simulink model "chloro_m"  (Simulink 7.9)
settings: Solver=ode45  SolverMode=SingleTasking  StartTime=0.0  StopTime=999999  MaxStep=10  RelTol=1e-3  AbsTol=1e-3
values from neighbouring files (symbols this model uses):
  U = st_Varia('LongNames')    [chloro_i.m]
  x0 = [1 0 0]    [chloro_i.m]    (also in chloro_s.m = x0)
undefined symbols (not defined in the file or in its folder): B
settings Model: Creator=M.Sparnaaij  LastModifiedBy=M.Sparnaaij
settings DataIOCC: LimitDataPoints=off  SaveOutput=off  SaveTime=off  SignalLoggingName=sigsOut
settings OptimizationCC: BooleanDataType=off
settings DebuggingCC: SaveWithParameterizedLinksMsg=none  SignalResolutionControl=TryResolveAllWithWarning  SolverPrmCheckMsg=none  MultiTaskDSMMsg=warning  MultiTaskCondExecSysMsg=none  FcnCallInpInsideContextMsg=Use local settings  StrictBusMsg=None
settings HardwareCC: TargetUnknown=on
settings RTWCC: IncludeERTFirstTime=on
settings GRTTargetCC: CombineOutputUpdateFcns=off  GRTInterface=on

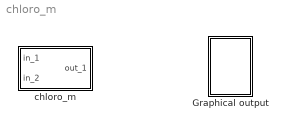
== system chloro_m ==
  Graphical output : Subsystem
      settings: OpenFcn=chloro_g
      mask Display:
      | plot(0,0,100,100,[80,20,20],[20,20,80],[80,69,60,52,45,39,33,28,24,20],[65,65,64,61,57,52,45,37,30,20])
      | disp('');
      | text(100,100,'chloro', 'horizontalAlignment', 'right', 'verticalAlignment', 'top');
  chloro_m : Subsystem  Description=chloro
      mask init:
      | filenaam='.\StimelaData\chloro_p.mat';
      | 
      | [Pn,Fn,Fext]=Fileprop(filenaam);
      | 
      | errstr = st_UniqName(filenaam,'filenaam=''','SubSystem','OpenFcn');
      | if errstr, error([errstr 'The filename "' filenaam '" is already in use. Choose a different filename.']), end
      | 
      | P = chloro_p(filenaam);
      | [B,x0,U]=chloro_i(filenaam);
      | V = st_Varia;
      settings: OpenFcn=|
      | filenaam='.\StimelaData\chloro_p.mat';
      | st_ParameterInput('init',gcb,filenaam,'chloro');
      mask Display:
      | plot(0,0,100,100,[0 20],[85 85],[0 20],[80 80],[0 20],[20 20],[80 100],[ 50 50],[80 100],[ 55 55],[20 80 80 20 20],[10 10 90  90 10]);
      | disp('')
      | text(50,50,'chloro', 'horizontalAlignment', 'center', 'verticalAlignment', 'middle');
      | text(50,0,Fn, 'horizontalAlignment', 'center', 'verticalAlignment', 'base');

== system chloro_m/Graphical output ==
  note: plotten

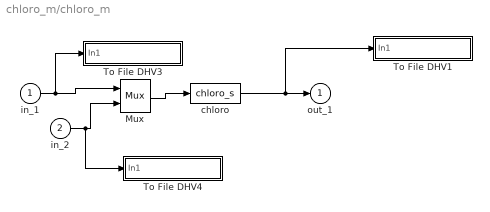
== system chloro_m/chloro_m ==
  in_1 : Inport
  in_2 : Inport  Port=2
  Mux : Mux  Inputs=[U.Number B.Setpoints]
  To File DHV1 : Subsystem  mask(To File DHV){naam=[filenaam(1:length(filenaam)-4) '_out.sti']}
      mask prompts: naam "Naam van bestand"
      mask init:
      | set_param([gcb '/To File'],'Filename',naam);
      mask Display: disp(naam)
  To File DHV3 : Subsystem  mask(To File DHV){naam=[filenaam(1:length(filenaam)-4) '_in.sti']}
      mask prompts: naam "Naam van bestand"
      mask init:
      | set_param([gcb '/To File'],'Filename',naam);
      mask Display: disp(naam)
  To File DHV4 : Subsystem  mask(To File DHV){naam=[filenaam(1:length(filenaam)-4) '_ES.sti']}
      mask prompts: naam "Naam van bestand"
      mask init:
      | set_param([gcb '/To File'],'Filename',naam);
      mask Display: disp(naam)
  chloro : S-Function  FunctionName=chloro_s  Parameters=B,x0,U,P  EnableBusSupport=off
  out_1 : Outport  InitialOutput=0
  wires:
  chloro/1 -> out_1/1, To File DHV1/1(In1)
  Mux/1 -> chloro/1
  in_1/1 -> Mux/1, To File DHV3/1(In1)
  in_2/1 -> Mux/2, To File DHV4/1(In1)

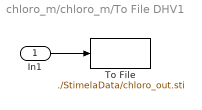
== system chloro_m/chloro_m/To File DHV1 ==
  In1 : Inport
  To File : ToFile  Filename=./StimelaData/chloro_out.sti  MatrixName=chloroout
  wires:
  In1/1 -> To File/1

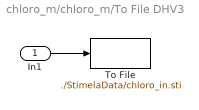
== system chloro_m/chloro_m/To File DHV3 ==
  In1 : Inport
  To File : ToFile  Filename=./StimelaData/chloro_in.sti  MatrixName=chloroin
  wires:
  In1/1 -> To File/1

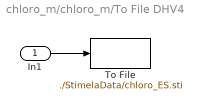
== system chloro_m/chloro_m/To File DHV4 ==
  In1 : Inport
  To File : ToFile  Filename=./StimelaData/chloro_ES.sti  MatrixName=chloroES
  wires:
  In1/1 -> To File/1
